simulink model "reset_integrator"  (R2018b)
settings: Solver=FixedStepAuto  StartTime=0.0  StopTime=10.0  FixedStep=1e-3  RelTol=1e-3
undefined symbols (not defined in the file or in its folder): DiscIntNeverNeededParam
libraries: simulink x1
settings Model: Creator=User  LastModifiedBy=wout7

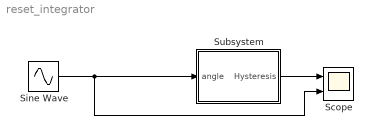
== system reset_integrator ==
  Scope : Scope  NumInputPorts=2
  Sine Wave : Sin  Amplitude=20  SampleTime=0
  Subsystem : Subsystem
  wires:
  Subsystem/1(Hysteresis) -> Scope/1
  Sine Wave/1 -> Scope/2, Subsystem/1(angle)

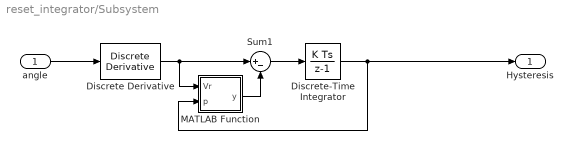
== system reset_integrator/Subsystem ==
  angle : Inport
  Discrete Derivative : simulink/Discrete/Discrete Derivative  gainval=1.0  ICPrevScaledInput=0.0  OutMin=[]  OutMax=[]  OutDataType=fixdt(1, 16)  OutScaling=2^-10  DoSatur=off
  Discrete-Time Integrator : DiscreteIntegrator  SampleTime=-1  ICPrevOutput=DiscIntNeverNeededParam  ICPrevScaledInput=DiscIntNeverNeededParam
  MATLAB Function : MATLAB Function  TreatAsAtomicUnit=on
  Sum1 : Sum  Inputs=|+-
  Hysteresis : Outport
  wires:
  MATLAB Function/1(y) -> Sum1/2
  angle/1 -> Discrete Derivative/1
  Sum1/1 -> Discrete-Time Integrator/1
  Discrete Derivative/1 -> Sum1/1, MATLAB Function/1(Vr)
  Discrete-Time Integrator/1 -> Hysteresis/1, MATLAB Function/2(p)

== matlab function reset_integrator/Subsystem/MATLAB Function ==
  data: Vr input; y output; p input
function y = fcn(Vr,p)
if Vr>0 && p>=17
    y = Vr;
elseif Vr<0 && p<=-17
    y = Vr;
else
    y = 0;
end
